simulink model "masa_resorte_amortiguador_sin_mask"  (R2024a)
settings: Solver=VariableStepAuto  StartTime=0.0  StopTime=10.0  RelTol=1e-3
model workspace (MAT data in the model file):
  b = 0.8
  k1 = 1.5
  k2 = 2
  m1 = 2
  m2 = 1

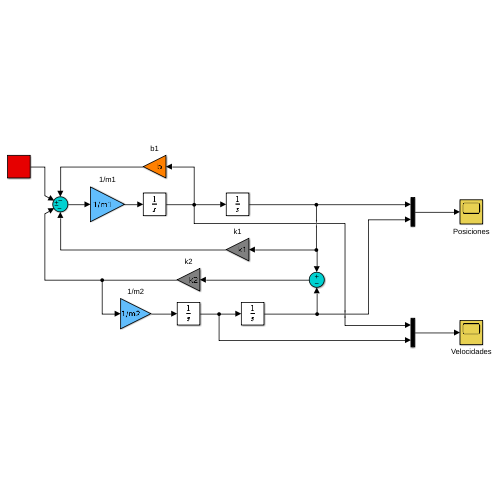
[thumbnail: Simulink's stored preview of the top-level diagram]
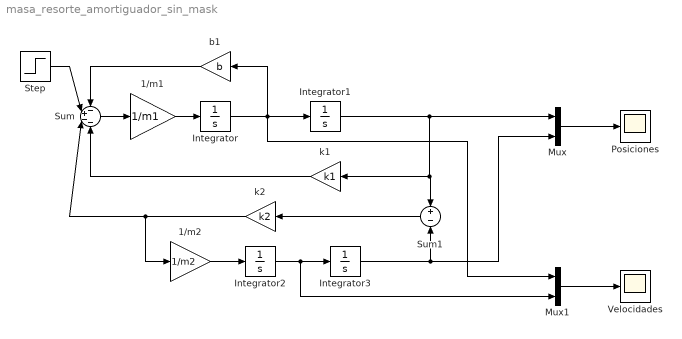
== system masa_resorte_amortiguador_sin_mask ==
  1/m1 : Gain  Gain=1/m1
  1/m2 : Gain  Gain=1/m2
  Integrator{,1..3} (4 alike) : Integrator
  Mux : Mux  Inputs=2
  Mux1 : Mux  Inputs=2
  Posiciones : Scope
  Step : Step  SampleTime=0
  Sum : Sum  Inputs=-+--
  Sum1 : Sum  Inputs=+|-
  Velocidades : Scope
  b1 : Gain  Gain=b
  k1 : Gain  Gain=k1
  k2 : Gain  Gain=k2
  wires:
  1/m1/1 -> Integrator/1
  1/m2/1 -> Integrator2/1
  Sum/1 -> 1/m1/1
  b1/1 -> Sum/1
  k1/1 -> Sum/4
  Sum1/1 -> k2/1
  k2/1 -> Sum/3, 1/m2/1
  Step/1 -> Sum/2
  Integrator1/1 -> Mux/1, Sum1/1, k1/1
  Integrator3/1 -> Sum1/2, Mux/2
  Mux/1 -> Posiciones/1
  Mux1/1 -> Velocidades/1
  Integrator2/1 -> Mux1/2, Integrator3/1
  Integrator/1 -> Mux1/1, b1/1, Integrator1/1
